simulink model "ComissionamentoMesa"  (R2024a)
settings: Solver=FixedStepAuto  StartTime=0.0  StopTime=inf  FixedStep=1e-3  RelTol=1e-3
model workspace (MAT data in the model file):
  mdlWSDbList = ["tramontina_database_curtis.dbc" "tramontina_database_curtis_mesa.dbc"]
undefined symbols (not defined in the file): Down, flap_front_left_down, flap_front_left_up, flap_front_right_down, flap_front_right_up, flap_rear_left_down, flap_rear_left_up, flap_rear_right_down, flap_rear_right_up, Pull
libraries: speedgoatlib_IO60X_IO69X x5, tramontina_database_curtis_mesalib x5, tramontina_database_curtislib x1, speedgoatlib_IO691 x1
settings Model: Creator=anderson.bordin  LastModifiedBy=matlab.cut
settings SolverCC: ConcurrentTasks=on  PositivePriorityOrder=on
settings OptimizationCC: BlockReduction=off  OptimizeBlockIOStorage=off
settings DebuggingCC: TasksWithSamePriorityMsg=none
settings HardwareCC: ProdBitPerLong=64  ProdLongLongMode=on  ProdHWDeviceType=Intel->x86-64 (Linux 64)
settings RTWCC: Description=Speedgoat Real-Time Target Machine  SystemTargetFile=speedgoat.tlc  TemplateMakefile=slrealtime_default_tmf  Toolchain=Simulink Real-Time Toolchain  BuildConfiguration=Faster Runs  CodeExecutionProfiling=on  TargetLang=C++
settings CodeAppCC: ForceParamTrailComments=on  MaxIdLength=127
settings SimulinkRealTimeTargetCC: InstructionSetFMA=off  LogToMDFFile=off

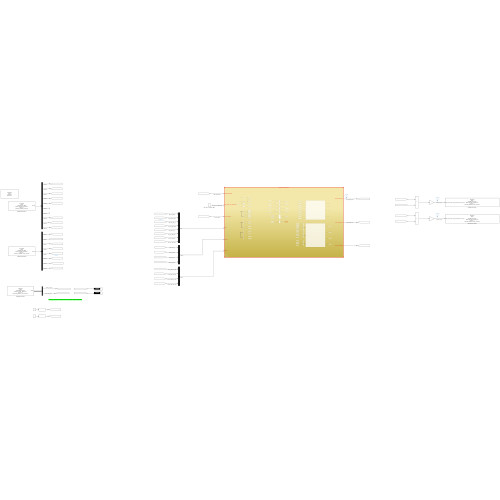
[thumbnail: Simulink's stored preview of the top-level diagram]
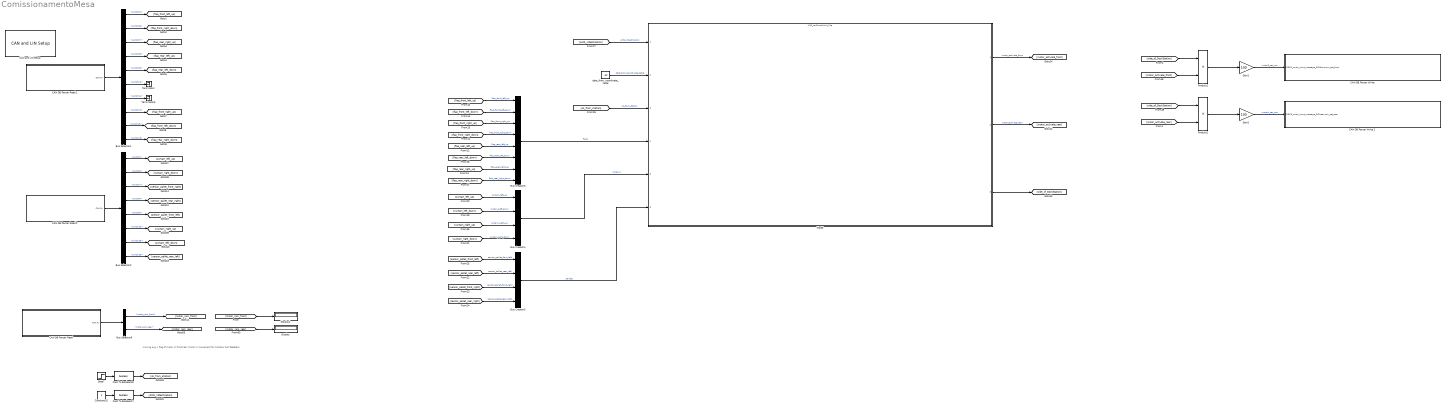
== system ComissionamentoMesa ==
  note: moving avg + flag of motor in front/rear motor in movement for CANbus IHM feedback
  Bus Creator3 : BusCreator  Inputs=flap_front_left_up,flap_front_left_down,flap_front_right_up,flap_front_right_down,flap_rear_left_up,flap_rear_left_down,flap_rear_right_up,flap_rear_right_down  OutDataTypeStr=Bus: IOs_flaps_bool
  Bus Creator4 : BusCreator  Inputs=4
  Bus Creator5 : BusCreator  Inputs=4
  Bus Selector1 : BusSelector  OutputSignals=ID934_curtis_encoder_left.switch01,ID934_curtis_encoder_left.switch06,ID934_curtis_encoder_left.switch07,ID934_curtis_encoder_left.switch08,ID934_curtis_encoder_left.switch09,ID934_curtis_encoder_left.switch10,ID934_curtis_encoder_left.switch12,ID934_curtis_encoder_left.switch13,ID934_curtis_encoder_left.switch15,ID934_curtis_encoder_left.switch18
  Bus Selector2 : BusSelector  OutputSignals=ID936_curtis_encoder_RCUfront.switch1,ID936_curtis_encoder_RCUfront.switch6,ID936_curtis_encoder_RCUfront.switch7,ID936_curtis_encoder_RCUfront.switch8,ID936_curtis_encoder_RCUfront.switch9,ID936_curtis_encoder_RCUfront.switch13,ID936_curtis_encoder_RCUfront.switch15,ID936_curtis_encoder_RCUfront.switch18
  Bus Selector6 : BusSelector  OutputSignals=ID424_curtis_feedback_message_RCUfront.motor_rpm_front,ID425_curtis_feedback_message_RCUrear.motor_rpm_rear
  "CAN DB Parser Read " : Subsystem
      settings: OpenFcn=sg_can.OpenFcnRead;
      mask Help: eval('sg.utils.help.show(''io_main/refentry_ref_can_ofa_parsing_read'');')
      mask Display: disp('Speedgoat\nIO691\nCAN DB Parser Read\nModule ID: IO691 - Module ID 1\nChannel:  1\ntramontina_database_curtis_mesa.dbc ');
  CAN DB Parser Read 1 : Subsystem
      settings: OpenFcn=sg_can.OpenFcnRead;
      mask Help: eval('sg.utils.help.show(''io_main/refentry_ref_can_ofa_parsing_read'');')
      mask Display: disp('Speedgoat\nIO691\nCAN DB Parser Read\nModule ID: IO691 - Module ID 1\nChannel:  1\ntramontina_database_curtis.dbc ');
  CAN DB Parser Read 2 : Subsystem
      settings: OpenFcn=sg_can.OpenFcnRead;
      mask Help: eval('sg.utils.help.show(''io_main/refentry_ref_can_ofa_parsing_read'');')
      mask Display: disp('Speedgoat\nIO691\nCAN DB Parser Read\nModule ID: IO691 - Module ID 1\nChannel:  1\ntramontina_database_curtis_mesa.dbc ');
  "CAN DB Parser Write " : Subsystem
      settings: OpenFcn=sg_can.OpenFcnWrite;
      mask Help: eval('sg.utils.help.show(''io_main/refentry_ref_can_ofa_parsing_write'');')
      mask Display: disp('Speedgoat\nIO691\nCAN DB Parser Write\nModule ID: IO691 - Module ID 1\nChannel:  1\ntramontina_database_curtis_mesa.dbc ');
  CAN DB Parser Write 2 : Subsystem
      settings: OpenFcn=sg_can.OpenFcnWrite;
      mask Help: eval('sg.utils.help.show(''io_main/refentry_ref_can_ofa_parsing_write'');')
      mask Display: disp('Speedgoat\nIO691\nCAN DB Parser Write\nModule ID: IO691 - Module ID 1\nChannel:  1\ntramontina_database_curtis_mesa.dbc ');
  "CAN and LIN Setup " : speedgoatlib_IO691/CAN and LIN Setup   moduleInitValues="[691    1    1   -1   -1]"  id=1  moduleType=IO691  pciSlot=-1  canChn1=CAN (HS)  canChn2=Disabled  canChn3=Disabled  canChn4=Disabled  linChn1=Disabled  linChn2=Disabled  canInitStructArray=[]  canTermStructArray=[]  gpioChnx=Disabled  canChn1InitValues="[2   2   8   1  16   3  19   2   2   5   2   0]"  arbBdrChn1=500 kBaud  clockDividerChn1=Enable  arbManBdrChn1=[8,1,16,3]  fdBdrChn1=5.0 MBaud  fdManBdrChn1=[2,2,5,2]  termResistor1=off  canChn2InitValues="[1   0   4   1  16   3  19   2   2   5   2   0]"  arbBdrChn2=1.0 MBaud  clockDividerChn2=Enable  arbManBdrChn2=[4,1,16,3]  fdBdrChn2=5.0 MBaud  fdManBdrChn2=[2,2,5,2]  termResistor2=off  canChn3InitValues="[1   0   2   8  31   8  19   2   2   5   2   0]"  arbBdrChn3=1.0 MBaud  clockDividerChn3=Enable  arbManBdrChn3=[2,8,31,8]  fdBdrChn3=5.0 MBaud  fdManBdrChn3=[2,2,5,2]  termResistor3=off  canChn4InitValues="[1   0   2   8  31   8  19   2   2   5   2   0]"  arbBdrChn4=1.0 MBaud  clockDividerChn4=Enable  arbManBdrChn4=[2,8,31,8]  fdBdrChn4=5.0 MBaud  fdManBdrChn4=[2,2,5,2]  termResistor4=off  linChn1InitValues="[0  9600]"  linBtrChn1=9600  linChn2InitValues="[0  9600]"  linBtrChn2=9600  doInitTermStruct="[0  5  0  0  0]"  parDoChannels=[1 2]  parDoVoltage=5  parDoInitValues=0  parDoReset=1  parNumOfDoS=0  parDiChannels=[3 4]  parDiVoltage=5  parDiPull=Pull-Down
      settings: SourceProductName=IO691
  Cast To Boolean17 : DataTypeConversion  OutDataTypeStr=boolean  SaturateOnIntegerOverflow=off  RndMeth=Floor
  Cast To Boolean20 : DataTypeConversion  OutDataTypeStr=boolean  SaturateOnIntegerOverflow=off  RndMeth=Floor
  Constant15 : Constant
  Display : Display
  Display1 : Display
  Gain1 : Gain  Gain=100
  Gain2 : Gain  Gain=100
  Model : ModelReference  ModelNameDialog=AMR_rcuControlUnit_24a.slx  SimulationMode=Normal  ModelReferenceVersion=1.7
  Product1 : Product
  Product2 : Product
  Step7 : Step  Time=15.5
  Terminator : Terminator
  Terminator5 : Terminator
  data_from_coordinate_table : Constant  Value=-12
  wires:
  "CAN DB Parser Read "/1(CAN Rx) -> Bus Selector6/1
  Bus Selector6/1 -> [motor_rpm_front]  "<motor_rpm_front>"
  CAN DB Parser Read 1/1(CAN Rx) -> Bus Selector1/1
  CAN DB Parser Read 2/1(CAN Rx) -> Bus Selector2/1
  Bus Selector1/6 -> Terminator/1  "<switch10>"
  Bus Selector1/5 -> [flap_rear_left_down]  "<switch09>"
  Bus Selector1/8 -> [flap_front_right_up]  "<switch13>"
  Bus Selector1/9 -> [flap_front_left_down]  "<switch15>"
  Bus Selector1/10 -> [flap_rear_right_down]  "<switch18>"
  Bus Selector1/1 -> [flap_front_left_up]  "<switch01>"
  Bus Selector1/2 -> [flap_front_right_down]  "<switch06>"
  Bus Selector1/3 -> [flap_rear_right_up]  "<switch07>"
  Bus Selector1/4 -> [flap_rear_left_up]  "<switch08>"
  Bus Selector1/7 -> Terminator5/1  "<switch12>"
  Bus Selector2/7 -> [curtain_left_down]  "<switch15>"
  Bus Selector2/1 -> [curtain_left_up]  "<switch1>"
  Bus Selector2/2 -> [curtain_right_down]  "<switch6>"
  Bus Selector2/3 -> [sensor_pallet_front_right]  "<switch7>"
  Bus Selector2/4 -> [sensor_pallet_rear_right]  "<switch8>"
  Bus Selector2/5 -> [sensor_pallet_front_left]  "<switch9>"
  Bus Selector2/6 -> [curtain_right_up]  "<switch13>"
  Bus Selector2/8 -> [sensor_pallet_rear_left]  "<switch18>"
  [side_of_DockStation] -> Product1/1
  Gain1/1 -> "CAN DB Parser Write "/1(ID552_curtis_input_message_RCUfront.rpm_set_front)  "motor3_set_rpm"
  [motor_activate_rear] -> Product2/2
  Gain2/1 -> CAN DB Parser Write 2/1(ID553_curtis_input_message_RCUrear.rpm_set_rear)  "motor4_set_rpm"
  [side_of_DockStation] -> Product2/1
  Product1/1 -> Gain1/1
  Product2/1 -> Gain2/1
  Bus Selector6/2 -> [motor_rpm_rear]  "<motor_rpm_rear>"
  [motor_activate_front] -> Product1/2
  [motor_rpm_front] -> Display1/1
  [motor_rpm_rear] -> Display/1
  [sensor_pallet_front_right] -> Bus Creator5/3  "sensor_pallet_front_right"
  [curtain_right_down] -> Bus Creator4/4  "curtain_right_down"
  [flap_rear_left_up] -> Bus Creator3/5  "flap_rear_left_up"
  [curtain_right_up] -> Bus Creator4/3  "curtain_right_up"
  [sensor_pallet_rear_left] -> Bus Creator5/2  "sensor_pallet_rear_left"
  [curtain_left_down] -> Bus Creator4/2  "curtain_left_down"
  [sensor_pallet_front_left] -> Bus Creator5/1  "sensor_pallet_front_left"
  [flap_rear_right_up] -> Bus Creator3/7  "flap_rear_right_up"
  [flap_front_left_up] -> Bus Creator3/1  "flap_front_left_up"
  [flap_front_right_down] -> Bus Creator3/4  "flap_front_right_down"
  [flap_rear_left_down] -> Bus Creator3/6  "flap_rear_left_down"
  [curtain_left_up] -> Bus Creator4/1  "curtain_left_up"
  [flap_rear_right_down] -> Bus Creator3/8  "flap_rear_right_down"
  [flap_front_left_down] -> Bus Creator3/2  "flap_front_left_down"
  [sensor_pallet_rear_right] -> Bus Creator5/4  "sensor_pallet_rear_right"
  [flap_front_right_up] -> Bus Creator3/3  "flap_front_right_up"
  Bus Creator3/1 -> Model/4  "flaps"
  Step7/1 -> Cast To Boolean20/1
  Cast To Boolean20/1 -> [ok_from_station]
  [ok_from_station] -> Model/3  "ok_from_station"
  [AMR_inDestination] -> Model/1  "AMR_inDestination"
  data_from_coordinate_table/1 -> Model/2  "data_from_coordinate_table"
  Cast To Boolean17/1 -> [AMR_inDestination]
  Constant15/1 -> Cast To Boolean17/1
  Model/2 -> [motor_activate_rear]  "motor_activate_rear"
  Model/1 -> [motor_activate_front]  "motor_activate_front"
  Model/3 -> [side_of_DockStation]
  Bus Creator4/1 -> Model/5  "curtains"
  Bus Creator5/1 -> Model/6  "pallets"

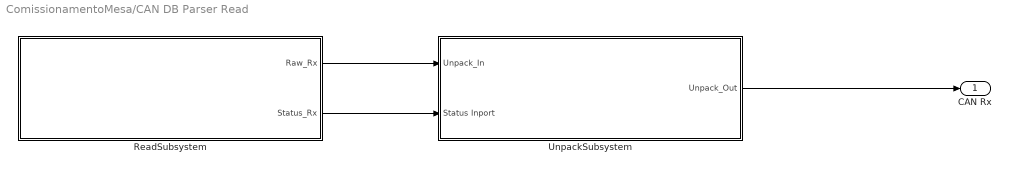
== system ComissionamentoMesa/CAN DB Parser Read  ==
  ReadSubsystem : Subsystem
  UnpackSubsystem : Subsystem
  CAN Rx : Outport
  wires:
  ReadSubsystem/1(Raw_Rx) -> UnpackSubsystem/1(Unpack_In)
  ReadSubsystem/2(Status_Rx) -> UnpackSubsystem/2(Status Inport)
  UnpackSubsystem/1(Unpack_Out) -> CAN Rx/1

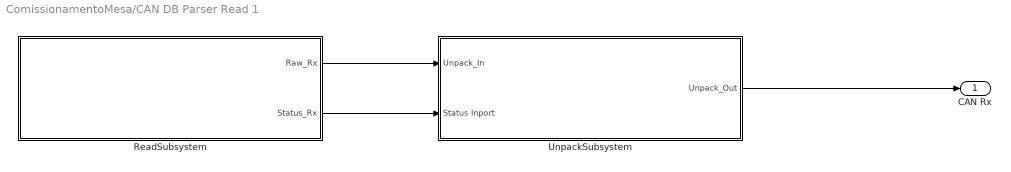
== system ComissionamentoMesa/CAN DB Parser Read 1 ==
  ReadSubsystem : Subsystem
  UnpackSubsystem : Subsystem
  CAN Rx : Outport
  wires:
  ReadSubsystem/1(Raw_Rx) -> UnpackSubsystem/1(Unpack_In)
  ReadSubsystem/2(Status_Rx) -> UnpackSubsystem/2(Status Inport)
  UnpackSubsystem/1(Unpack_Out) -> CAN Rx/1

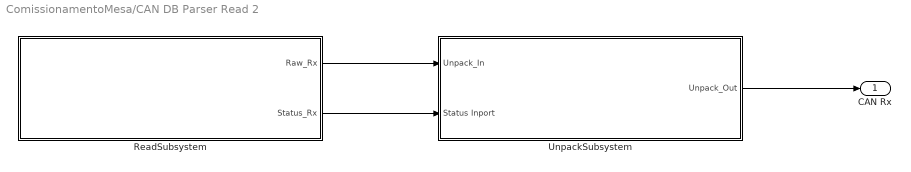
== system ComissionamentoMesa/CAN DB Parser Read 2 ==
  ReadSubsystem : Subsystem
  UnpackSubsystem : Subsystem
  CAN Rx : Outport
  wires:
  ReadSubsystem/1(Raw_Rx) -> UnpackSubsystem/1(Unpack_In)
  ReadSubsystem/2(Status_Rx) -> UnpackSubsystem/2(Status Inport)
  UnpackSubsystem/1(Unpack_Out) -> CAN Rx/1

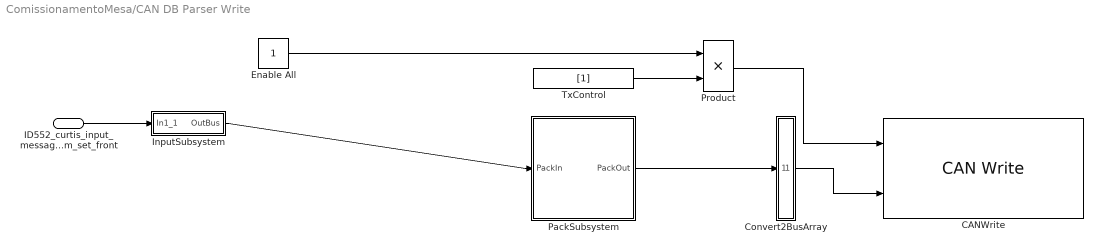
== system ComissionamentoMesa/CAN DB Parser Write  ==
  ID552_curtis_input_message_RCUfront.rpm_set_front : Inport
  CANWrite : speedgoatlib_IO60X_IO69X/CAN/CAN Write   moduleType=IO691  id=1  channel=1  canType=CAN (HS)  messageType=CAN (HS)  useBusIn=on  numOfMsg=1  enableInput=on  enableStatusPort=off  ts=-1  initValues=[691 1 -1 0 1 1 0 1 1 1]
  Convert2BusArray : Subsystem
  Enable All : Constant  OutDataTypeStr=boolean
  InputSubsystem : Subsystem
  PackSubsystem : Subsystem
  Product : Product  OutDataTypeStr=uint32
  TxControl : Constant  Value=[1]  OutDataTypeStr=uint32
  wires:
  PackSubsystem/1(PackOut) -> Convert2BusArray/1(InBus)
  Convert2BusArray/1(BusArrayOut) -> CANWrite/2
  Product/1 -> CANWrite/1
  TxControl/1 -> Product/2
  Enable All/1 -> Product/1
  ID552_curtis_input_message_RCUfront.rpm_set_front/1 -> InputSubsystem/1(In1_1)
  InputSubsystem/1(OutBus) -> PackSubsystem/1(PackIn)

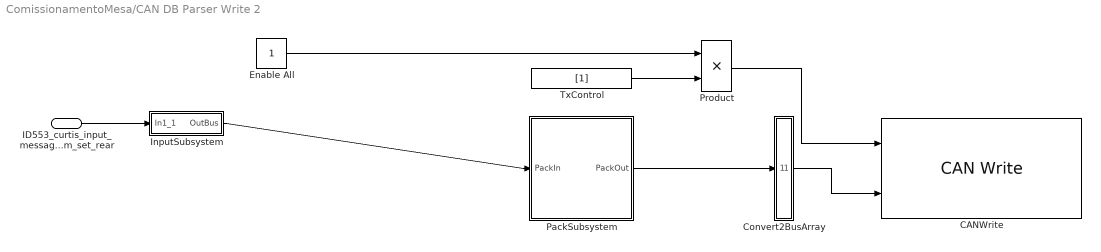
== system ComissionamentoMesa/CAN DB Parser Write 2 ==
  ID553_curtis_input_message_RCUrear.rpm_set_rear : Inport
  CANWrite : speedgoatlib_IO60X_IO69X/CAN/CAN Write   moduleType=IO691  id=1  channel=1  canType=CAN (HS)  messageType=CAN (HS)  useBusIn=on  numOfMsg=1  enableInput=on  enableStatusPort=off  ts=-1  initValues=[691 1 -1 0 1 1 0 1 1 1]
  Convert2BusArray : Subsystem
  Enable All : Constant  OutDataTypeStr=boolean
  InputSubsystem : Subsystem
  PackSubsystem : Subsystem
  Product : Product  OutDataTypeStr=uint32
  TxControl : Constant  Value=[1]  OutDataTypeStr=uint32
  wires:
  PackSubsystem/1(PackOut) -> Convert2BusArray/1(InBus)
  Convert2BusArray/1(BusArrayOut) -> CANWrite/2
  Product/1 -> CANWrite/1
  TxControl/1 -> Product/2
  Enable All/1 -> Product/1
  ID553_curtis_input_message_RCUrear.rpm_set_rear/1 -> InputSubsystem/1(In1_1)
  InputSubsystem/1(OutBus) -> PackSubsystem/1(PackIn)

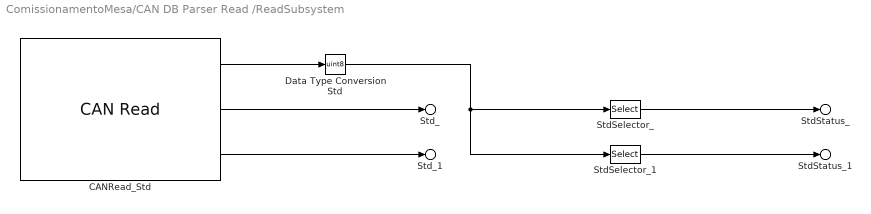
== system ComissionamentoMesa/CAN DB Parser Read /ReadSubsystem ==
  CANRead_Std : speedgoatlib_IO60X_IO69X/CAN/CAN Read   moduleType=IO691  id=1  channel=1  canType=CAN (HS)  messageType=CAN (HS)  useBusOut=on  HasMulRead=Specify by IDs  MsgIDlist="[424  425]"  isEFF=off  LabelInHex=off  enableInput=off  initValues=[691 1 -1 0 1 1 0 1 2 0 2 424 425]  ts=-1
  Data Type ConversionStd : DataTypeConversion  OutDataTypeStr=uint8  SaturateOnIntegerOverflow=off  RndMeth=Floor
  StdSelector_ : Selector  IndexOptions=Index vector (dialog)  Indices=1  OutputSizes=1
  StdSelector_1 : Selector  IndexOptions=Index vector (dialog)  Indices=2  OutputSizes=1
  Std_ : Outport  PortName=Raw_Rx  Element=Std.ID424
  Std_1 : Outport  PortName=Raw_Rx  Element=Std.ID425
  StdStatus_ : Outport  Port=2  PortName=Status_Rx  Element=Std.ID424
  StdStatus_1 : Outport  Port=2  PortName=Status_Rx  Element=Std.ID425
  wires:
  CANRead_Std/1 -> Data Type ConversionStd/1
  CANRead_Std/2 -> Std_/1
  CANRead_Std/3 -> Std_1/1
  Data Type ConversionStd/1 -> StdSelector_/1, StdSelector_1/1
  StdSelector_/1 -> StdStatus_/1
  StdSelector_1/1 -> StdStatus_1/1

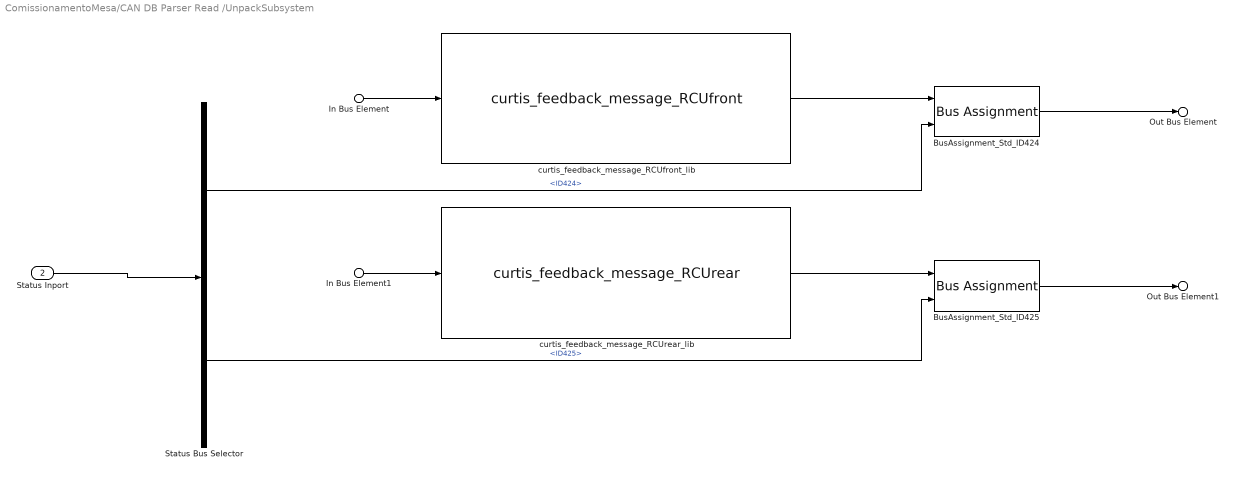
== system ComissionamentoMesa/CAN DB Parser Read /UnpackSubsystem ==
  In Bus Element : Inport  PortName=Unpack_In  Element=Std.ID424
  In Bus Element1 : Inport  PortName=Unpack_In  Element=Std.ID425
  Status Inport : Inport  Port=2
  BusAssignment_Std_ID424 : BusAssignment  AssignedSignals=MessageStatus.Status
  BusAssignment_Std_ID425 : BusAssignment  AssignedSignals=MessageStatus.Status
  Status Bus Selector : BusSelector  OutputSignals=Std.ID424,Std.ID425
  curtis_feedback_message_RCUfront_lib : tramontina_database_curtis_mesalib/CAN unpack/curtis_feedback_message_RCUfront  SystemSampleTime=-1  VariantActivationTime=update diagram  AllowFlexibleInterface=on  Latency=0  AutoFrameSizeCalculation=off
  curtis_feedback_message_RCUrear_lib : tramontina_database_curtis_mesalib/CAN unpack/curtis_feedback_message_RCUrear  SystemSampleTime=-1  VariantActivationTime=update diagram  AllowFlexibleInterface=on  Latency=0  AutoFrameSizeCalculation=off
  Out Bus Element : Outport  PortName=Unpack_Out  Element=ID424_curtis_feedback_message_RCUfront
  Out Bus Element1 : Outport  PortName=Unpack_Out  Element=ID425_curtis_feedback_message_RCUrear
  wires:
  In Bus Element/1 -> curtis_feedback_message_RCUfront_lib/1
  curtis_feedback_message_RCUfront_lib/1 -> BusAssignment_Std_ID424/1
  BusAssignment_Std_ID424/1 -> Out Bus Element/1
  In Bus Element1/1 -> curtis_feedback_message_RCUrear_lib/1
  curtis_feedback_message_RCUrear_lib/1 -> BusAssignment_Std_ID425/1
  BusAssignment_Std_ID425/1 -> Out Bus Element1/1
  Status Inport/1 -> Status Bus Selector/1
  Status Bus Selector/1 -> BusAssignment_Std_ID424/2  "<ID424>"
  Status Bus Selector/2 -> BusAssignment_Std_ID425/2  "<ID425>"

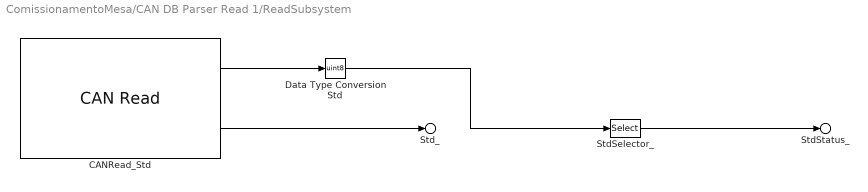
== system ComissionamentoMesa/CAN DB Parser Read 1/ReadSubsystem ==
  CANRead_Std : speedgoatlib_IO60X_IO69X/CAN/CAN Read   moduleType=IO691  id=1  channel=1  canType=CAN (HS)  messageType=CAN (HS)  useBusOut=on  HasMulRead=Specify by IDs  MsgIDlist=[934]  isEFF=off  LabelInHex=off  enableInput=off  initValues=[691 1 -1 0 1 1 0 1 2 0 1 934]  ts=-1
  Data Type ConversionStd : DataTypeConversion  OutDataTypeStr=uint8  SaturateOnIntegerOverflow=off  RndMeth=Floor
  StdSelector_ : Selector  IndexOptions=Index vector (dialog)  Indices=1  OutputSizes=1
  Std_ : Outport  PortName=Raw_Rx  Element=Std.ID934
  StdStatus_ : Outport  Port=2  PortName=Status_Rx  Element=Std.ID934
  wires:
  CANRead_Std/1 -> Data Type ConversionStd/1
  CANRead_Std/2 -> Std_/1
  Data Type ConversionStd/1 -> StdSelector_/1
  StdSelector_/1 -> StdStatus_/1

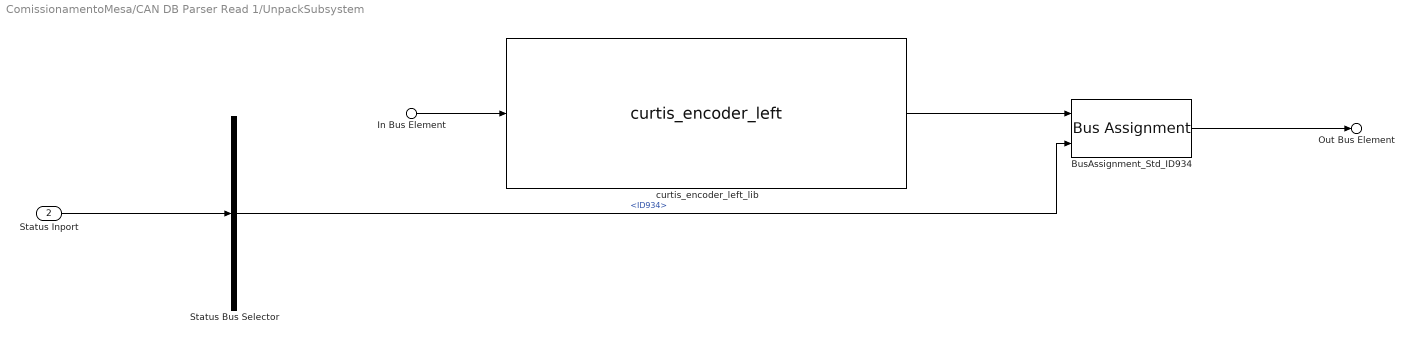
== system ComissionamentoMesa/CAN DB Parser Read 1/UnpackSubsystem ==
  In Bus Element : Inport  PortName=Unpack_In  Element=Std.ID934
  Status Inport : Inport  Port=2
  BusAssignment_Std_ID934 : BusAssignment  AssignedSignals=MessageStatus.Status
  Status Bus Selector : BusSelector  OutputSignals=Std.ID934
  curtis_encoder_left_lib : tramontina_database_curtislib/CAN unpack/curtis_encoder_left  SystemSampleTime=-1  VariantActivationTime=update diagram  AllowFlexibleInterface=on  Latency=0  AutoFrameSizeCalculation=off
  Out Bus Element : Outport  PortName=Unpack_Out  Element=ID934_curtis_encoder_left
  wires:
  In Bus Element/1 -> curtis_encoder_left_lib/1
  curtis_encoder_left_lib/1 -> BusAssignment_Std_ID934/1
  BusAssignment_Std_ID934/1 -> Out Bus Element/1
  Status Inport/1 -> Status Bus Selector/1
  Status Bus Selector/1 -> BusAssignment_Std_ID934/2  "<ID934>"

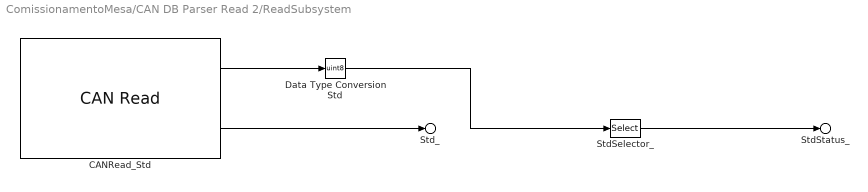
== system ComissionamentoMesa/CAN DB Parser Read 2/ReadSubsystem ==
  CANRead_Std : speedgoatlib_IO60X_IO69X/CAN/CAN Read   moduleType=IO691  id=1  channel=1  canType=CAN (HS)  messageType=CAN (HS)  useBusOut=on  HasMulRead=Specify by IDs  MsgIDlist=[936]  isEFF=off  LabelInHex=off  enableInput=off  initValues=[691 1 -1 0 1 1 0 1 2 0 1 936]  ts=-1
  Data Type ConversionStd : DataTypeConversion  OutDataTypeStr=uint8  SaturateOnIntegerOverflow=off  RndMeth=Floor
  StdSelector_ : Selector  IndexOptions=Index vector (dialog)  Indices=1  OutputSizes=1
  Std_ : Outport  PortName=Raw_Rx  Element=Std.ID936
  StdStatus_ : Outport  Port=2  PortName=Status_Rx  Element=Std.ID936
  wires:
  CANRead_Std/1 -> Data Type ConversionStd/1
  CANRead_Std/2 -> Std_/1
  Data Type ConversionStd/1 -> StdSelector_/1
  StdSelector_/1 -> StdStatus_/1

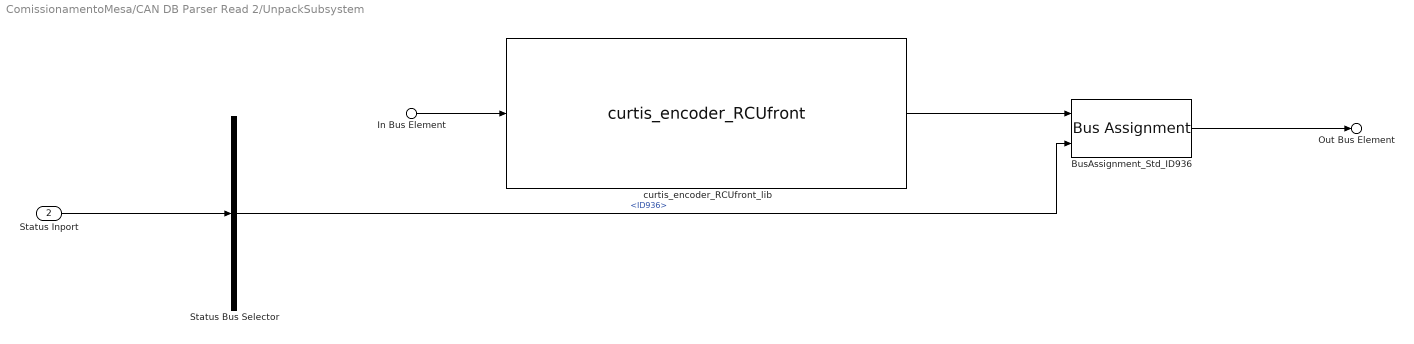
== system ComissionamentoMesa/CAN DB Parser Read 2/UnpackSubsystem ==
  In Bus Element : Inport  PortName=Unpack_In  Element=Std.ID936
  Status Inport : Inport  Port=2
  BusAssignment_Std_ID936 : BusAssignment  AssignedSignals=MessageStatus.Status
  Status Bus Selector : BusSelector  OutputSignals=Std.ID936
  curtis_encoder_RCUfront_lib : tramontina_database_curtis_mesalib/CAN unpack/curtis_encoder_RCUfront  SystemSampleTime=-1  VariantActivationTime=update diagram  AllowFlexibleInterface=on  Latency=0  AutoFrameSizeCalculation=off
  Out Bus Element : Outport  PortName=Unpack_Out  Element=ID936_curtis_encoder_RCUfront
  wires:
  In Bus Element/1 -> curtis_encoder_RCUfront_lib/1
  curtis_encoder_RCUfront_lib/1 -> BusAssignment_Std_ID936/1
  BusAssignment_Std_ID936/1 -> Out Bus Element/1
  Status Inport/1 -> Status Bus Selector/1
  Status Bus Selector/1 -> BusAssignment_Std_ID936/2  "<ID936>"

== system ComissionamentoMesa/CAN DB Parser Write /Convert2BusArray ==
  In1 : Inport  PortName=InBus  Element=ID552_curtis_input_message_RCUfront
  BusArray : Concatenate  NumInputs=1
  BusArrayOut : Outport
  wires:
  In1/1 -> BusArray/1
  BusArray/1 -> BusArrayOut/1

== system ComissionamentoMesa/CAN DB Parser Write /InputSubsystem ==
  In1_1 : Inport
  ID552_curtis_input_message_RCUfront.rpm_set_front : Outport  PortName=OutBus  Element=ID552_curtis_input_message_RCUfront.rpm_set_front
  wires:
  In1_1/1 -> ID552_curtis_input_message_RCUfront.rpm_set_front/1

== system ComissionamentoMesa/CAN DB Parser Write /PackSubsystem ==
  In Bus Element : Inport  PortName=PackIn  Element=ID552_curtis_input_message_RCUfront
  curtis_input_message_RCUfront_lib : tramontina_database_curtis_mesalib/CAN pack/curtis_input_message_RCUfront  SystemSampleTime=-1  VariantActivationTime=update diagram  AllowFlexibleInterface=on  Latency=0  AutoFrameSizeCalculation=off
  In Bus Element1 : Outport  PortName=PackOut  Element=ID552_curtis_input_message_RCUfront
  wires:
  In Bus Element/1 -> curtis_input_message_RCUfront_lib/1
  curtis_input_message_RCUfront_lib/1 -> In Bus Element1/1

== system ComissionamentoMesa/CAN DB Parser Write 2/Convert2BusArray ==
  In1 : Inport  PortName=InBus  Element=ID553_curtis_input_message_RCUrear
  BusArray : Concatenate  NumInputs=1
  BusArrayOut : Outport
  wires:
  In1/1 -> BusArray/1
  BusArray/1 -> BusArrayOut/1

== system ComissionamentoMesa/CAN DB Parser Write 2/InputSubsystem ==
  In1_1 : Inport
  ID553_curtis_input_message_RCUrear.rpm_set_rear : Outport  PortName=OutBus  Element=ID553_curtis_input_message_RCUrear.rpm_set_rear
  wires:
  In1_1/1 -> ID553_curtis_input_message_RCUrear.rpm_set_rear/1

== system ComissionamentoMesa/CAN DB Parser Write 2/PackSubsystem ==
  In Bus Element : Inport  PortName=PackIn  Element=ID553_curtis_input_message_RCUrear
  curtis_input_message_RCUrear_lib : tramontina_database_curtis_mesalib/CAN pack/curtis_input_message_RCUrear  SystemSampleTime=-1  VariantActivationTime=update diagram  AllowFlexibleInterface=on  Latency=0  AutoFrameSizeCalculation=off
  In Bus Element1 : Outport  PortName=PackOut  Element=ID553_curtis_input_message_RCUrear
  wires:
  In Bus Element/1 -> curtis_input_message_RCUrear_lib/1
  curtis_input_message_RCUrear_lib/1 -> In Bus Element1/1
